simulink model "DiscreteModelGroundVeicle"  (R2020b)
settings: Solver=VariableStepAuto  StartTime=0.0  StopTime=10.0  RelTol=1e-3
values from neighbouring files (symbols this model uses):
  x0 = [1;1;0]    [initialization.m]
undefined symbols (not defined in the file or in its folder): sigbuilder_block
settings Model: Creator=joaolourenco  LastModifiedBy=joaolourenco

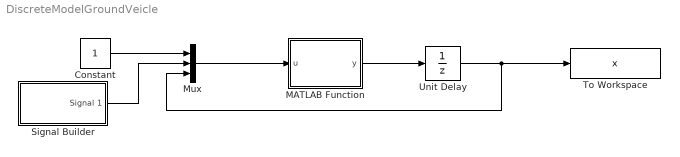
== system DiscreteModelGroundVeicle ==
  Constant : Constant
  MATLAB Function : MATLAB Function  TreatAsAtomicUnit=on
  Mux : Mux  Inputs=3
  Signal Builder : Subsystem  Tag=STV Subsys  LoadFcn=sigbuilder_block('load');  StartFcn=sigbuilder_block('start');  StopFcn=sigbuilder_block('stop');  ClipboardFcn=sigbuilder_block('clipboard');  mask(Sigbuilder block){tuvar=[0:10]}
      mask help: Simulink:masks:SigbuilderBlock_MD
      mask init:
      | if ~strcmp(get_param(bdroot(gcbh),'SimulationStatus'),'stopped') tuvar = sigbuilder_block('maskInit'); end
      settings: CopyFcn=sigbuilder_block('copy');  DeleteFcn=sigbuilder_block('delete');  ModelCloseFcn=sigbuilder_block('modelClose');  PreSaveFcn=sigbuilder_block('preSave');  PauseFcn=sigbuilder_block('pause');  ContinueFcn=sigbuilder_block('continue');  NameChangeFcn=sigbuilder_block('namechange');  OpenFcn=sigbuilder_block('open',[434.526 191.368 550.105 400.421 ]);  CloseFcn=sigbuilder_block('close');
      mask Display: plot(0, 0, 100, 100,[2, 2, 32, 32, 2], [68, 8, 8, 68, 68],[32, 2], [38, 38], [32, 19, 2],[53, 60, 44], [32, 17, 17, 2],[16, 16, 31, 31]);txt = getActiveGroup(gcbh);text(2, 100, txt,'verticalAlignment', 'top');
  To Workspace : ToWorkspace  VariableName=x  SampleTime=-1
  Unit Delay : UnitDelay  InitialCondition=x0  SampleTime=0.1  HasFrameUpgradeWarning=on
  wires:
  MATLAB Function/1(y) -> Unit Delay/1
  Mux/1 -> MATLAB Function/1(u)
  Unit Delay/1 -> To Workspace/1, Mux/3
  Constant/1 -> Mux/1
  Signal Builder/1(Signal 1) -> Mux/2

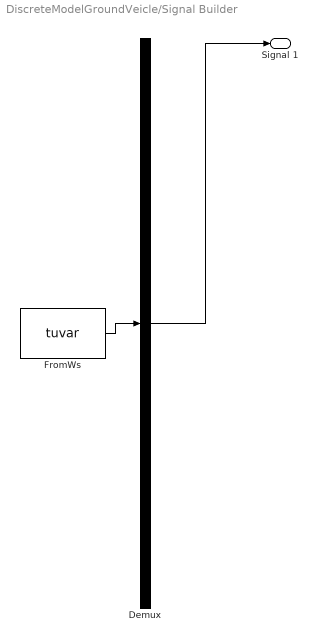
== system DiscreteModelGroundVeicle/Signal Builder ==
  Demux : Demux  Tag=STV Demux  Outputs=1
      settings: DisplayOption=none
  FromWs : FromWorkspace  Tag=STV FromWs  VariableName=tuvar
      SigBuilderData=|
      | common.afterFinalStr = 'Extrapolate'
      | common.sampleTime = 0
      | dataSet.timeRange = [0 10]
      | dataSet.name = 'Group 1'
      | sbobj.Groups.Name = 'Group 1'
      | sbobj.Groups.Signals.Name = 'Signal 1'
      | sbobj.Groups.Signals.XData = [0 4 4 6 6 10]
      | sbobj.Groups.Signals.YData = [0 0 1 1 0 0]
  Signal 1 : Outport  Tag=STV Outport
  wires:
  Demux/1 -> Signal 1/1
  FromWs/1 -> Demux/1

== matlab function DiscreteModelGroundVeicle/MATLAB Function ==
  data: u input; y output
function y = fcn(u)

% parse u and define v1, v2, and x
v1 = u(1);
v2 = u(2);
x1 = u(3);
x2 = u(4);
x3 = u(5);

% parameters
d = 0.01;
c = 0.1;

%definitiong of G
x1plus = x1 + d * sin(x3) * v1;
x2plus = x2 + d * cos(x3) * v1;
x3plus = x3 + c * v2;

y = [x1plus; x2plus; x3plus;];
